simulink model "vcmultex"  (Simulink 3.00)
settings: Solver=FixedStepDiscrete  StartTime=0.0  StopTime=10.0  RelTol=1e-3
undefined symbols (not defined in the file or in its folder): j
libraries: smxl x1
settings Model: LastModifiedBy=giampiero

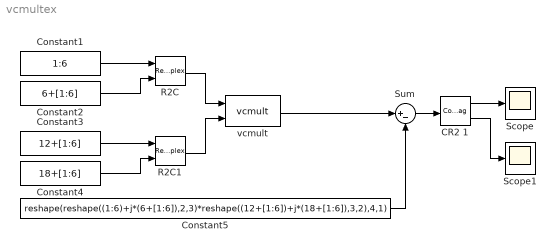
== system vcmultex ==
  CR2 1 : ComplexToRealImag  Output=RealAndImag
  Constant1 : Constant  Value=1:6
  Constant2 : Constant  Value=6+[1:6]
  Constant3 : Constant  Value=12+[1:6]
  Constant4 : Constant  Value=18+[1:6]
  Constant5 : Constant  Value=reshape(reshape((1:6)+j*(6+[1:6]),2,3)*reshape((12+[1:6])+j*(18+[1:6]),3,2),4,1)
  R2C : RealImagToComplex  Input=RealAndImag  ConstantPart=0
  R2C1 : RealImagToComplex  Input=RealAndImag  ConstantPart=0
  Scope : Scope
      settings: TimeRange=10  YMin=-4e-015  YMax=4e-015  SaveToWorkspace=off  SaveName=ScopeData
  Scope1 : Scope
      settings: TimeRange=10  YMin=-4e-015  YMax=4e-015  SaveToWorkspace=off  SaveName=ScopeData
  Sum : Sum  Inputs=|+-  SaturateOnIntegerOverflow=on
  vcmult : smxl/Complex Matrices/vcmult  d=[2 3 2]
  wires:
  R2C/1 -> vcmult/1
  vcmult/1 -> Sum/1
  Constant1/1 -> R2C/1
  Constant3/1 -> R2C1/1
  Constant2/1 -> R2C/2
  Constant4/1 -> R2C1/2
  Sum/1 -> CR2 1/1
  CR2 1/1 -> Scope/1
  CR2 1/2 -> Scope1/1
  Constant5/1 -> Sum/2
  R2C1/1 -> vcmult/2
